simulink model "System_Theta_Space"  (R2019b)
settings: Solver=VariableStepAuto  StartTime=0.0  StopTime=10  FixedStep=.001  MaxStep=.001  RelTol=1e-6  EnableMultiTasking=on
values from neighbouring files (symbols this model uses):
  Kd = [75;75;75;40;1;1]    [SimRun_ThetaSpace.m]
  Ki = [0;500;300;300;0;0]    [SimRun_ThetaSpace.m]
  Kp = [500;500;500;300;10;10]    [SimRun_ThetaSpace.m]
undefined symbols (not defined in the file or in its folder): DiscIntNeverNeededParam
(part 1 of 4)
settings Model: Creator=Andrew Petruska  LastModifiedBy=Andrew Petruska
settings DataIOCC: ReturnWorkspaceOutputs=off
settings OptimizationCC: LifeSpan=inf
settings DebuggingCC: SFUnexpectedBacktrackingDiag=warning  SFNoUnconditionalDefaultTransitionDiag=warning  ArithmeticOperatorsInVariantConditions=warning
settings SFSimCC: SimUseLocalCustomCode=off  CustomCodeUndefinedFunction=UseInterfaceOnly
settings RTWCC: RTWUseLocalCustomCode=off
settings CodeAppCC: StateflowObjectComments=on
settings GRTTargetCC: TargetLangStandard=C89/C90 (ANSI)  GeneratePreprocessorConditionals=Disable all
settings ConfigComp: CovMetricSettings=dw  CovHtmlReporting=on  CovSaveCumulativeToWorkspaceVar=on  CovSaveSingleToWorkspaceVar=on  CovExternalEMLEnable=off

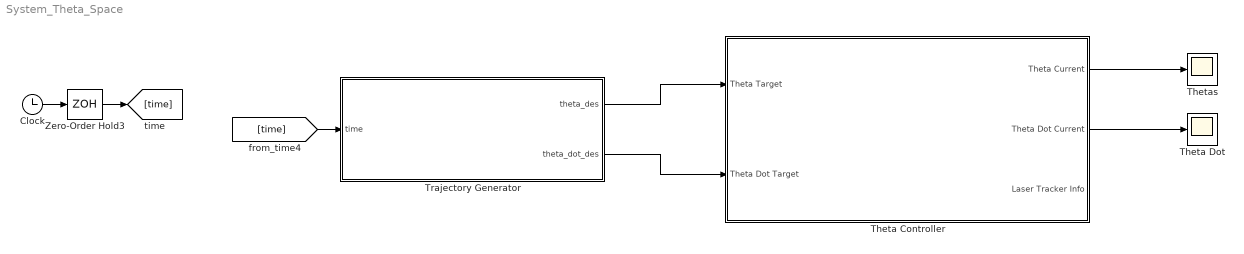
== system System_Theta_Space ==
  Clock : Clock
  Theta Controller : Subsystem
  Theta Dot : Scope
  Thetas : Scope
  Trajectory Generator : MATLAB Function  TreatAsAtomicUnit=on
  Zero-Order Hold3 : ZeroOrderHold  SampleTime=0.001
  wires:
  Clock/1 -> Zero-Order Hold3/1
  Zero-Order Hold3/1 -> [time]
  [time] -> Trajectory Generator/1(time)
  Theta Controller/1(Theta Current) -> Thetas/1
  Theta Controller/2(Theta Dot Current) -> Theta Dot/1
  Trajectory Generator/1(theta_des) -> Theta Controller/1(Theta Target)
  Trajectory Generator/2(theta_dot_des) -> Theta Controller/2(Theta Dot Target)

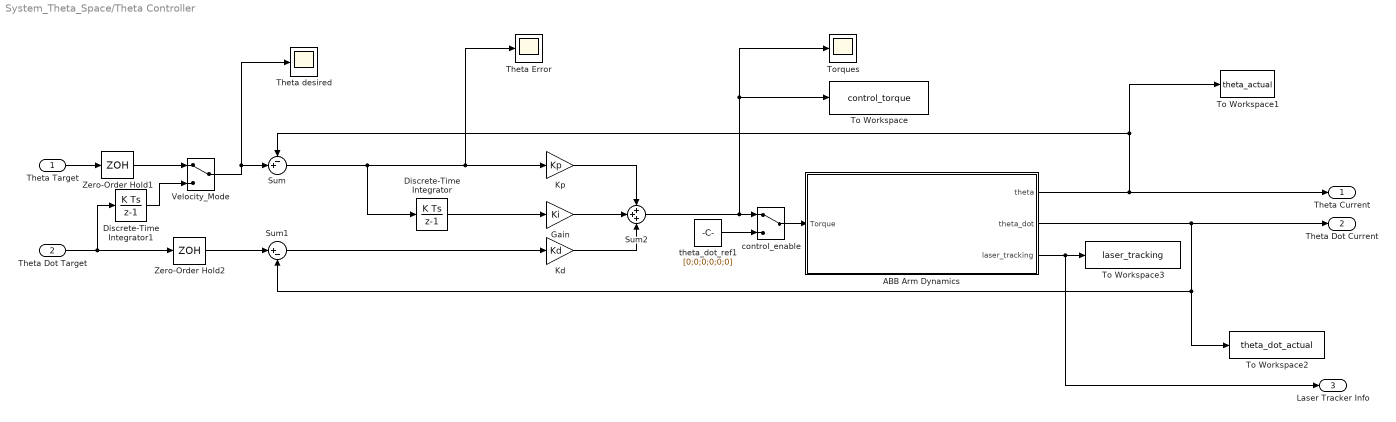
== system System_Theta_Space/Theta Controller ==
  Theta Target : Inport
  Theta Dot Target : Inport  Port=2
  ABB Arm Dynamics : Subsystem
  Discrete-Time Integrator : DiscreteIntegrator  gainval=1  SampleTime=-1  ICPrevOutput=DiscIntNeverNeededParam  ICPrevScaledInput=DiscIntNeverNeededParam
  Discrete-Time Integrator1 : DiscreteIntegrator  gainval=1  SampleTime=-1  ICPrevOutput=DiscIntNeverNeededParam  ICPrevScaledInput=DiscIntNeverNeededParam
  Gain : Gain  Gain=Ki
  Kd : Gain  Gain=Kd
  Kp : Gain  Gain=Kp
  Sum : Sum  Inputs=-+|
  Sum1 : Sum  Inputs=|+-
  Sum2 : Sum  Inputs=+++
  Theta Error : Scope
  Theta desired : Scope
  To Workspace : ToWorkspace  VariableName=control_torque  SaveFormat=Structure With Time  SampleTime=-1
  To Workspace1 : ToWorkspace  VariableName=theta_actual  SaveFormat=Structure With Time  SampleTime=-1
  To Workspace2 : ToWorkspace  VariableName=theta_dot_actual  SaveFormat=Structure With Time  SampleTime=-1
  To Workspace3 : ToWorkspace  VariableName=laser_tracking  SaveFormat=Structure With Time  SampleTime=-1
  Torques : Scope
  Velocity_Mode : ManualSwitch
  Zero-Order Hold1 : ZeroOrderHold  SampleTime=0.001
  Zero-Order Hold2 : ZeroOrderHold  SampleTime=0.001
  control_enable : ManualSwitch
  theta_dot_ref1 : Constant  Value=[0;0;0;0;0;0]
  Theta Current : Outport
  Theta Dot Current : Outport  Port=2
  Laser Tracker Info : Outport  Port=3
  wires:
  control_enable/1 -> ABB Arm Dynamics/1(Torque)
  ABB Arm Dynamics/1(theta) -> Sum/1, To Workspace1/1, Theta Current/1
  Sum/1 -> Discrete-Time Integrator/1, Theta Error/1, Kp/1
  ABB Arm Dynamics/2(theta_dot) -> Sum1/2, To Workspace2/1, Theta Dot Current/1
  Sum2/1 -> To Workspace/1, Torques/1, control_enable/1
  Discrete-Time Integrator/1 -> Gain/1
  theta_dot_ref1/1 -> control_enable/2
  ABB Arm Dynamics/3(laser_tracking) -> Laser Tracker Info/1, To Workspace3/1
  Sum1/1 -> Kd/1
  Kp/1 -> Sum2/1
  Gain/1 -> Sum2/2
  Kd/1 -> Sum2/3
  Theta Target/1 -> Zero-Order Hold1/1
  Theta Dot Target/1 -> Discrete-Time Integrator1/1, Zero-Order Hold2/1
  Zero-Order Hold2/1 -> Sum1/1
  Velocity_Mode/1 -> Theta desired/1, Sum/2
  Zero-Order Hold1/1 -> Velocity_Mode/1
  Discrete-Time Integrator1/1 -> Velocity_Mode/2

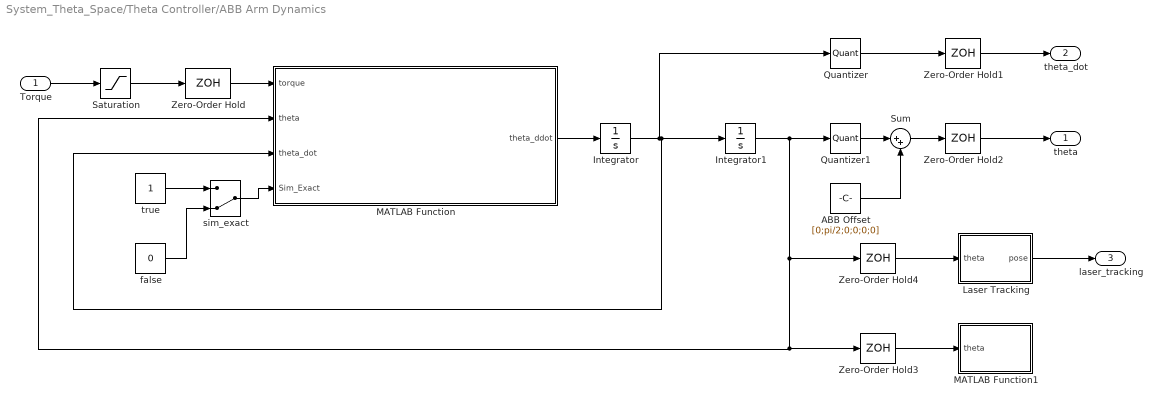
== system System_Theta_Space/Theta Controller/ABB Arm Dynamics ==
  Torque : Inport
  ABB Offset : Constant  Value=[0;pi/2;0;0;0;0]
  Integrator : Integrator  InitialCondition=zeros(6,1)
  Integrator1 : Integrator  InitialCondition=zeros(6,1)
  Laser Tracking : MATLAB Function  TreatAsAtomicUnit=on
  MATLAB Function : MATLAB Function  TreatAsAtomicUnit=on
  MATLAB Function1 : MATLAB Function  TreatAsAtomicUnit=on
  Quantizer : Quantizer  QuantizationInterval=1/2^32
  Quantizer1 : Quantizer  QuantizationInterval=1/2^32
  Saturation : Saturate  UpperLimit=350  LowerLimit=-350
  Sum : Sum  Inputs=|++
  Zero-Order Hold{,1..2,4} (4 alike) : ZeroOrderHold  SampleTime=0.001
  Zero-Order Hold3 : ZeroOrderHold  SampleTime=.05
  false : Constant  Value=0
  sim_exact : ManualSwitch  CurrentSetting=0
  true : Constant
  theta : Outport
  theta_dot : Outport  Port=2
  laser_tracking : Outport  Port=3
  wires:
  Torque/1 -> Saturation/1
  MATLAB Function/1(theta_ddot) -> Integrator/1
  Integrator/1 -> Quantizer/1, MATLAB Function/3(theta_dot), Integrator1/1
  Zero-Order Hold/1 -> MATLAB Function/1(torque)
  Quantizer/1 -> Zero-Order Hold1/1
  Zero-Order Hold1/1 -> theta_dot/1
  Zero-Order Hold2/1 -> theta/1
  Integrator1/1 -> Quantizer1/1, MATLAB Function/2(theta), Zero-Order Hold3/1, Zero-Order Hold4/1
  Zero-Order Hold3/1 -> MATLAB Function1/1(theta)
  Sum/1 -> Zero-Order Hold2/1
  Quantizer1/1 -> Sum/1
  ABB Offset/1 -> Sum/2
  Laser Tracking/1(pose) -> laser_tracking/1
  Saturation/1 -> Zero-Order Hold/1
  Zero-Order Hold4/1 -> Laser Tracking/1(theta)
  sim_exact/1 -> MATLAB Function/4(Sim_Exact)
  true/1 -> sim_exact/1
  false/1 -> sim_exact/2

== matlab function System_Theta_Space/Theta Controller/ABB Arm Dynamics/MATLAB Function1 ==
  data: theta input
function drawArm(theta)
%#codegen
coder.extrinsic('evalin');
coder.extrinsic('load');
persistent figNum axisHandel Sim_Exact points3D drawCSM sizeCSM;

if isempty(Sim_Exact)
    Sim_Exact = evalin('base','Sim_Exact');
    sizeCSM = 1;
    sizeCSM = evalin('base','sizeCSM');
    drawCSM = evalin('base','drawCSM');
    points3D = zeros(sizeCSM,3,'double');
    
    if drawCSM
        %a.points3D = zeros(sizeCSM,3,'double');
        a = struct('points3D',points3D);
        a = load('points3D.mat','points3D');
        points3D = a.points3D;
    end
end

th1 = theta(1);
th2 = theta(2);
th3 = theta(3);
th4 = theta(4);
th5 = theta(5);
th6 = theta(6);

if(Sim_Exact)
    
    T06 = [ sin(th6)*(cos(th4)*sin(th1) + sin(th4)*(cos(th1)*sin(th2)*sin(th3) - cos(th1)*cos(th2)*cos(th3))) + cos(th6)*(cos(th5)*(sin(th1)*sin(th4) - cos(th4)*(cos(th1)*sin(th2)*sin(th3) - cos(th1)*cos(th2)*cos(th3))) - sin(th5)*(cos(th1)*cos(th2)*sin(th3) + cos(th1)*cos(th3)*sin(th2))), cos(th6)*(cos(th4)*sin(th1) + sin(th4)*(cos(th1)*sin(th2)*sin(th3) - cos(th1)*cos(th2)*cos(th3))) - sin(th6)*(cos(th5)*(sin(th1)*sin(th4) - cos(th4)*(cos(th1)*sin(th2)*sin(th3) - cos(th1)*cos(th2)*cos(th3))) - sin(th5)*(cos(th1)*cos(th2)*sin(th3) + cos(th1)*cos(th3)*sin(th2))), - sin(th5)*(sin(th1)*sin(th4) - cos(th4)*(cos(th1)*sin(th2)*sin(th3) - cos(th1)*cos(th2)*cos(th3))) - cos(th5)*(cos(th1)*cos(th2)*sin(th3) + cos(th1)*cos(th3)*sin(th2)), (27*cos(th1)*cos(th2))/100 - (9*sin(th5)*(sin(th1)*sin(th4) - cos(th4)*(cos(th1)*sin(th2)*sin(th3) - cos(th1)*cos(th2)*cos(th3))))/125 - (9*cos(th5)*(cos(th1)*cos(th2)*sin(th3) + cos(th1)*cos(th3)*sin(th2)))/125 - (7*cos(th1)*sin(th2)*sin(th3))/100 + (7*cos(th1)*cos(th2)*cos(th3))/100 - (151*cos(th1)*cos(th2)*sin(th3))/500 - (151*cos(th1)*cos(th3)*sin(th2))/500;
        - sin(th6)*(cos(th1)*cos(th4) - sin(th4)*(sin(th1)*sin(th2)*sin(th3) - cos(th2)*cos(th3)*sin(th1))) - cos(th6)*(cos(th5)*(cos(th1)*sin(th4) + cos(th4)*(sin(th1)*sin(th2)*sin(th3) - cos(th2)*cos(th3)*sin(th1))) + sin(th5)*(cos(th2)*sin(th1)*sin(th3) + cos(th3)*sin(th1)*sin(th2))), sin(th6)*(cos(th5)*(cos(th1)*sin(th4) + cos(th4)*(sin(th1)*sin(th2)*sin(th3) - cos(th2)*cos(th3)*sin(th1))) + sin(th5)*(cos(th2)*sin(th1)*sin(th3) + cos(th3)*sin(th1)*sin(th2))) - cos(th6)*(cos(th1)*cos(th4) - sin(th4)*(sin(th1)*sin(th2)*sin(th3) - cos(th2)*cos(th3)*sin(th1))), sin(th5)*(cos(th1)*sin(th4) + cos(th4)*(sin(th1)*sin(th2)*sin(th3) - cos(th2)*cos(th3)*sin(th1))) - cos(th5)*(cos(th2)*sin(th1)*sin(th3) + cos(th3)*sin(th1)*sin(th2)), (27*cos(th2)*sin(th1))/100 + (9*sin(th5)*(cos(th1)*sin(th4) + cos(th4)*(sin(th1)*sin(th2)*sin(th3) - cos(th2)*cos(th3)*sin(th1))))/125 - (9*cos(th5)*(cos(th2)*sin(th1)*sin(th3) + cos(th3)*sin(th1)*sin(th2)))/125 - (151*cos(th2)*sin(th1)*sin(th3))/500 - (151*cos(th3)*sin(th1)*sin(th2))/500 - (7*sin(th1)*sin(th2)*sin(th3))/100 + (7*cos(th2)*cos(th3)*sin(th1))/100;
        sin(th4)*sin(th6)*(cos(th2)*sin(th3) + cos(th3)*sin(th2)) - cos(th6)*(sin(th5)*(cos(th2)*cos(th3) - sin(th2)*sin(th3)) + cos(th4)*cos(th5)*(cos(th2)*sin(th3) + cos(th3)*sin(th2))), sin(th6)*(sin(th5)*(cos(th2)*cos(th3) - sin(th2)*sin(th3)) + cos(th4)*cos(th5)*(cos(th2)*sin(th3) + cos(th3)*sin(th2))) + cos(th6)*sin(th4)*(cos(th2)*sin(th3) + cos(th3)*sin(th2)), cos(th4)*sin(th5)*(cos(th2)*sin(th3) + cos(th3)*sin(th2)) - cos(th5)*(cos(th2)*cos(th3) - sin(th2)*sin(th3)), (151*sin(th2)*sin(th3))/500 - (151*cos(th2)*cos(th3))/500 - (7*cos(th2)*sin(th3))/100 - (7*cos(th3)*sin(th2))/100 - (27*sin(th2))/100 - (9*cos(th5)*(cos(th2)*cos(th3) - sin(th2)*sin(th3)))/125 + (9*cos(th4)*sin(th5)*(cos(th2)*sin(th3) + cos(th3)*sin(th2)))/125 + 29/100;
        0, 0, 0, 1];
    
    P1 =[ 0
        0
        0.29];
    P2 = [ 0.27*cos(th1)*cos(th2);
        0.27*cos(th2)*sin(th1);
        0.29 - 0.27*sin(th2)];
    P3 = [ 0.27*cos(th1)*cos(th2) - 0.07*cos(th1)*sin(th2)*sin(th3) + 0.07*cos(th1)*cos(th2)*cos(th3);
        0.27*cos(th2)*sin(th1) - 0.07*sin(th1)*sin(th2)*sin(th3) + 0.07*cos(th2)*cos(th3)*sin(th1);
        0.29 - 0.07*cos(th2)*sin(th3) - 0.07*cos(th3)*sin(th2) - 0.27*sin(th2)];
    
    P4 = [ 0.27*cos(th1)*cos(th2) - 0.07*cos(th1)*sin(th2)*sin(th3) + 0.07*cos(th1)*cos(th2)*cos(th3) - 0.302*cos(th1)*cos(th2)*sin(th3) - 0.302*cos(th1)*cos(th3)*sin(th2);
        0.27*cos(th2)*sin(th1) - 0.302*cos(th2)*sin(th1)*sin(th3) - 0.302*cos(th3)*sin(th1)*sin(th2) - 0.07*sin(th1)*sin(th2)*sin(th3) + 0.07*cos(th2)*cos(th3)*sin(th1);
        0.302*sin(th2)*sin(th3) - 0.302*cos(th2)*cos(th3) - 0.07*cos(th2)*sin(th3) - 0.07*cos(th3)*sin(th2) - 0.27*sin(th2) + 0.29];
    P5 = [ 0.27*cos(th1)*cos(th2) - 0.07*cos(th1)*sin(th2)*sin(th3) + 0.07*cos(th1)*cos(th2)*cos(th3) - 0.302*cos(th1)*cos(th2)*sin(th3) - 0.302*cos(th1)*cos(th3)*sin(th2)
        0.27*cos(th2)*sin(th1) - 0.302*cos(th2)*sin(th1)*sin(th3) - 0.302*cos(th3)*sin(th1)*sin(th2) - 0.07*sin(th1)*sin(th2)*sin(th3) + 0.07*cos(th2)*cos(th3)*sin(th1)
        0.302*sin(th2)*sin(th3) - 0.302*cos(th2)*cos(th3) - 0.07*cos(th2)*sin(th3) - 0.07*cos(th3)*sin(th2) - 0.27*sin(th2) + 0.29];
    
    P6 =[ 0.27*cos(th1)*cos(th2) - 0.07*cos(th1)*sin(th2)*sin(th3) - 0.072*sin(th1)*sin(th4)*sin(th5) + 0.07*cos(th1)*cos(th2)*cos(th3) - 0.302*cos(th1)*cos(th2)*sin(th3) - 0.302*cos(th1)*cos(th3)*sin(th2) - 0.072*cos(th1)*cos(th2)*cos(th5)*sin(th3) - 0.072*cos(th1)*cos(th3)*cos(th5)*sin(th2) - 0.072*cos(th1)*cos(th2)*cos(th3)*cos(th4)*sin(th5) + 0.072*cos(th1)*cos(th4)*sin(th2)*sin(th3)*sin(th5);
        0.27*cos(th2)*sin(th1) - 0.302*cos(th2)*sin(th1)*sin(th3) - 0.302*cos(th3)*sin(th1)*sin(th2) + 0.072*cos(th1)*sin(th4)*sin(th5) - 0.07*sin(th1)*sin(th2)*sin(th3) + 0.07*cos(th2)*cos(th3)*sin(th1) - 0.072*cos(th2)*cos(th5)*sin(th1)*sin(th3) - 0.072*cos(th3)*cos(th5)*sin(th1)*sin(th2) - 0.072*cos(th2)*cos(th3)*cos(th4)*sin(th1)*sin(th5) + 0.072*cos(th4)*sin(th1)*sin(th2)*sin(th3)*sin(th5);
        0.302*sin(th2)*sin(th3) - 0.302*cos(th2)*cos(th3) - 0.07*cos(th2)*sin(th3) - 0.07*cos(th3)*sin(th2) - 0.27*sin(th2) + 0.072*cos(th5)*sin(th2)*sin(th3) - 0.072*cos(th2)*cos(th3)*cos(th5) + 0.072*cos(th2)*cos(th4)*sin(th3)*sin(th5) + 0.072*cos(th3)*cos(th4)*sin(th2)*sin(th5) + 0.29];
    
else
    
    T06 = [ sin(th6)*(cos(th4)*sin(th1) + sin(th4)*(cos(th1)*sin(th2)*sin(th3) - cos(th1)*cos(th2)*cos(th3))) + cos(th6)*(cos(th5)*(sin(th1)*sin(th4) - cos(th4)*(cos(th1)*sin(th2)*sin(th3) - cos(th1)*cos(th2)*cos(th3))) - sin(th5)*(cos(th1)*cos(th2)*sin(th3) + cos(th1)*cos(th3)*sin(th2))), cos(th6)*(cos(th4)*sin(th1) + sin(th4)*(cos(th1)*sin(th2)*sin(th3) - cos(th1)*cos(th2)*cos(th3))) - sin(th6)*(cos(th5)*(sin(th1)*sin(th4) - cos(th4)*(cos(th1)*sin(th2)*sin(th3) - cos(th1)*cos(th2)*cos(th3))) - sin(th5)*(cos(th1)*cos(th2)*sin(th3) + cos(th1)*cos(th3)*sin(th2))), - sin(th5)*(sin(th1)*sin(th4) - cos(th4)*(cos(th1)*sin(th2)*sin(th3) - cos(th1)*cos(th2)*cos(th3))) - cos(th5)*(cos(th1)*cos(th2)*sin(th3) + cos(th1)*cos(th3)*sin(th2)), (151838081588107*cos(th1)*cos(th2))/562949953421312 - (123928564092639*sin(th1))/72057594037927936 - (7184037743251309*cos(th1))/36893488147419103232 - (7330531551818703*cos(th4)*sin(th1))/36893488147419103232 - (5489399374888815*sin(th1)*sin(th4))/9223372036854775808 + (970893499285375*cos(th5)*(sin(th1)*sin(th4) - cos(th4)*(cos(th1)*sin(th2)*sin(th3) - cos(th1)*cos(th2)*cos(th3))))/9223372036854775808 - (5192391675427195*sin(th5)*(sin(th1)*sin(th4) - cos(th4)*(cos(th1)*sin(th2)*sin(th3) - cos(th1)*cos(th2)*cos(th3))))/72057594037927936 + (1663072680156839*sin(th6)*(cos(th4)*sin(th1) + sin(th4)*(cos(th1)*sin(th2)*sin(th3) - cos(th1)*cos(th2)*cos(th3))))/2305843009213693952 + (1663072680156839*cos(th6)*(cos(th5)*(sin(th1)*sin(th4) - cos(th4)*(cos(th1)*sin(th2)*sin(th3) - cos(th1)*cos(th2)*cos(th3))) - sin(th5)*(cos(th1)*cos(th2)*sin(th3) + cos(th1)*cos(th3)*sin(th2))))/2305843009213693952 + (5489399374888815*cos(th4)*(cos(th1)*sin(th2)*sin(th3) - cos(th1)*cos(th2)*cos(th3)))/9223372036854775808 - (5192391675427195*cos(th5)*(cos(th1)*cos(th2)*sin(th3) + cos(th1)*cos(th3)*sin(th2)))/72057594037927936 - (7330531551818703*sin(th4)*(cos(th1)*sin(th2)*sin(th3) - cos(th1)*cos(th2)*cos(th3)))/36893488147419103232 - (970893499285375*sin(th5)*(cos(th1)*cos(th2)*sin(th3) + cos(th1)*cos(th3)*sin(th2)))/9223372036854775808 - (1259578569946919*cos(th1)*sin(th2)*sin(th3))/18014398509481984 + (1259578569946919*cos(th1)*cos(th2)*cos(th3))/18014398509481984 - (5430591396830085*cos(th1)*cos(th2)*sin(th3))/18014398509481984 - (5430591396830085*cos(th1)*cos(th3)*sin(th2))/18014398509481984;
        - sin(th6)*(cos(th1)*cos(th4) - sin(th4)*(sin(th1)*sin(th2)*sin(th3) - cos(th2)*cos(th3)*sin(th1))) - cos(th6)*(cos(th5)*(cos(th1)*sin(th4) + cos(th4)*(sin(th1)*sin(th2)*sin(th3) - cos(th2)*cos(th3)*sin(th1))) + sin(th5)*(cos(th2)*sin(th1)*sin(th3) + cos(th3)*sin(th1)*sin(th2))), sin(th6)*(cos(th5)*(cos(th1)*sin(th4) + cos(th4)*(sin(th1)*sin(th2)*sin(th3) - cos(th2)*cos(th3)*sin(th1))) + sin(th5)*(cos(th2)*sin(th1)*sin(th3) + cos(th3)*sin(th1)*sin(th2))) - cos(th6)*(cos(th1)*cos(th4) - sin(th4)*(sin(th1)*sin(th2)*sin(th3) - cos(th2)*cos(th3)*sin(th1))), sin(th5)*(cos(th1)*sin(th4) + cos(th4)*(sin(th1)*sin(th2)*sin(th3) - cos(th2)*cos(th3)*sin(th1))) - cos(th5)*(cos(th2)*sin(th1)*sin(th3) + cos(th3)*sin(th1)*sin(th2)), (123928564092639*cos(th1))/72057594037927936 - (7184037743251309*sin(th1))/36893488147419103232 + (7330531551818703*cos(th1)*cos(th4))/36893488147419103232 + (151838081588107*cos(th2)*sin(th1))/562949953421312 + (5489399374888815*cos(th1)*sin(th4))/9223372036854775808 - (970893499285375*cos(th5)*(cos(th1)*sin(th4) + cos(th4)*(sin(th1)*sin(th2)*sin(th3) - cos(th2)*cos(th3)*sin(th1))))/9223372036854775808 + (5192391675427195*sin(th5)*(cos(th1)*sin(th4) + cos(th4)*(sin(th1)*sin(th2)*sin(th3) - cos(th2)*cos(th3)*sin(th1))))/72057594037927936 - (1663072680156839*sin(th6)*(cos(th1)*cos(th4) - sin(th4)*(sin(th1)*sin(th2)*sin(th3) - cos(th2)*cos(th3)*sin(th1))))/2305843009213693952 + (5489399374888815*cos(th4)*(sin(th1)*sin(th2)*sin(th3) - cos(th2)*cos(th3)*sin(th1)))/9223372036854775808 - (5192391675427195*cos(th5)*(cos(th2)*sin(th1)*sin(th3) + cos(th3)*sin(th1)*sin(th2)))/72057594037927936 - (1663072680156839*cos(th6)*(cos(th5)*(cos(th1)*sin(th4) + cos(th4)*(sin(th1)*sin(th2)*sin(th3) - cos(th2)*cos(th3)*sin(th1))) + sin(th5)*(cos(th2)*sin(th1)*sin(th3) + cos(th3)*sin(th1)*sin(th2))))/2305843009213693952 - (7330531551818703*sin(th4)*(sin(th1)*sin(th2)*sin(th3) - cos(th2)*cos(th3)*sin(th1)))/36893488147419103232 - (970893499285375*sin(th5)*(cos(th2)*sin(th1)*sin(th3) + cos(th3)*sin(th1)*sin(th2)))/9223372036854775808 - (5430591396830085*cos(th2)*sin(th1)*sin(th3))/18014398509481984 - (5430591396830085*cos(th3)*sin(th1)*sin(th2))/18014398509481984 - (1259578569946919*sin(th1)*sin(th2)*sin(th3))/18014398509481984 + (1259578569946919*cos(th2)*cos(th3)*sin(th1))/18014398509481984;
        sin(th4)*sin(th6)*(cos(th2)*sin(th3) + cos(th3)*sin(th2)) - cos(th6)*(sin(th5)*(cos(th2)*cos(th3) - sin(th2)*sin(th3)) + cos(th4)*cos(th5)*(cos(th2)*sin(th3) + cos(th3)*sin(th2))), sin(th6)*(sin(th5)*(cos(th2)*cos(th3) - sin(th2)*sin(th3)) + cos(th4)*cos(th5)*(cos(th2)*sin(th3) + cos(th3)*sin(th2))) + cos(th6)*sin(th4)*(cos(th2)*sin(th3) + cos(th3)*sin(th2)), cos(th4)*sin(th5)*(cos(th2)*sin(th3) + cos(th3)*sin(th2)) - cos(th5)*(cos(th2)*cos(th3) - sin(th2)*sin(th3)), (5430591396830085*sin(th2)*sin(th3))/18014398509481984 - (5430591396830085*cos(th2)*cos(th3))/18014398509481984 - (1259578569946919*cos(th2)*sin(th3))/18014398509481984 - (1259578569946919*cos(th3)*sin(th2))/18014398509481984 - (1663072680156839*cos(th6)*(sin(th5)*(cos(th2)*cos(th3) - sin(th2)*sin(th3)) + cos(th4)*cos(th5)*(cos(th2)*sin(th3) + cos(th3)*sin(th2))))/2305843009213693952 - (151838081588107*sin(th2))/562949953421312 + (5489399374888815*cos(th4)*(cos(th2)*sin(th3) + cos(th3)*sin(th2)))/9223372036854775808 - (5192391675427195*cos(th5)*(cos(th2)*cos(th3) - sin(th2)*sin(th3)))/72057594037927936 - (7330531551818703*sin(th4)*(cos(th2)*sin(th3) + cos(th3)*sin(th2)))/36893488147419103232 - (970893499285375*sin(th5)*(cos(th2)*cos(th3) - sin(th2)*sin(th3)))/9223372036854775808 - (970893499285375*cos(th4)*cos(th5)*(cos(th2)*sin(th3) + cos(th3)*sin(th2)))/9223372036854775808 + (5192391675427195*cos(th4)*sin(th5)*(cos(th2)*sin(th3) + cos(th3)*sin(th2)))/72057594037927936 + (1663072680156839*sin(th4)*sin(th6)*(cos(th2)*sin(th3) + cos(th3)*sin(th2)))/2305843009213693952 + 325695105792877/1125899906842624;
        0, 0, 0, 1];
    P1 = [ -0.000194724*cos(th1);
        -0.000194724*sin(th1);
        0.289275];
    P2 =[ 0.269719*cos(th1)*cos(th2) - 0.000812193*sin(th1) - 0.000194724*cos(th1);
        0.000812193*cos(th1) - 0.000194724*sin(th1) + 0.269719*cos(th2)*sin(th1);
        0.289275 - 0.269719*sin(th2)];
    P3 =[ 0.269719*cos(th1)*cos(th2) - 0.00171985*sin(th1) - 0.000194724*cos(th1) - 0.0699207*cos(th1)*sin(th2)*sin(th3) + 0.0699207*cos(th1)*cos(th2)*cos(th3);
        0.00171985*cos(th1) - 0.000194724*sin(th1) + 0.269719*cos(th2)*sin(th1) - 0.0699207*sin(th1)*sin(th2)*sin(th3) + 0.0699207*cos(th2)*cos(th3)*sin(th1);
        0.289275 - 0.0699207*cos(th2)*sin(th3) - 0.0699207*cos(th3)*sin(th2) - 0.269719*sin(th2)];
    
    P4 =[ 0.269719*cos(th1)*cos(th2) - 0.00171985*sin(th1) - 0.000194724*cos(th1) - 0.000595162*sin(th1)*sin(th4) - 0.0699207*cos(th1)*sin(th2)*sin(th3) + 0.0699207*cos(th1)*cos(th2)*cos(th3) - 0.301458*cos(th1)*cos(th2)*sin(th3) - 0.301458*cos(th1)*cos(th3)*sin(th2) - 0.000595162*cos(th1)*cos(th2)*cos(th3)*cos(th4) + 0.000595162*cos(th1)*cos(th4)*sin(th2)*sin(th3);
        0.00171985*cos(th1) - 0.000194724*sin(th1) + 0.269719*cos(th2)*sin(th1) + 0.000595162*cos(th1)*sin(th4) - 0.301458*cos(th2)*sin(th1)*sin(th3) - 0.301458*cos(th3)*sin(th1)*sin(th2) - 0.0699207*sin(th1)*sin(th2)*sin(th3) + 0.0699207*cos(th2)*cos(th3)*sin(th1) - 0.000595162*cos(th2)*cos(th3)*cos(th4)*sin(th1) + 0.000595162*cos(th4)*sin(th1)*sin(th2)*sin(th3);
        0.301458*sin(th2)*sin(th3) - 0.301458*cos(th2)*cos(th3) - 0.0699207*cos(th2)*sin(th3) - 0.0699207*cos(th3)*sin(th2) - 0.269719*sin(th2) + 0.000595162*cos(th2)*cos(th4)*sin(th3) + 0.000595162*cos(th3)*cos(th4)*sin(th2) + 0.289275];
    
    P5 = [ 0.269719*cos(th1)*cos(th2) - 0.00171985*sin(th1) - 0.000194724*cos(th1) - 0.000198694*cos(th4)*sin(th1) - 0.000595162*sin(th1)*sin(th4) - 0.0699207*cos(th1)*sin(th2)*sin(th3) + 0.000105264*cos(th5)*sin(th1)*sin(th4) + 0.0699207*cos(th1)*cos(th2)*cos(th3) - 0.301458*cos(th1)*cos(th2)*sin(th3) - 0.301458*cos(th1)*cos(th3)*sin(th2) - 0.000595162*cos(th1)*cos(th2)*cos(th3)*cos(th4) + 0.000198694*cos(th1)*cos(th2)*cos(th3)*sin(th4) + 0.000595162*cos(th1)*cos(th4)*sin(th2)*sin(th3) - 0.000105264*cos(th1)*cos(th2)*sin(th3)*sin(th5) - 0.000105264*cos(th1)*cos(th3)*sin(th2)*sin(th5) - 0.000198694*cos(th1)*sin(th2)*sin(th3)*sin(th4) + 0.000105264*cos(th1)*cos(th2)*cos(th3)*cos(th4)*cos(th5) - 0.000105264*cos(th1)*cos(th4)*cos(th5)*sin(th2)*sin(th3);
        0.00171985*cos(th1) - 0.000194724*sin(th1) + 0.000198694*cos(th1)*cos(th4) + 0.269719*cos(th2)*sin(th1) + 0.000595162*cos(th1)*sin(th4) - 0.301458*cos(th2)*sin(th1)*sin(th3) - 0.301458*cos(th3)*sin(th1)*sin(th2) - 0.0699207*sin(th1)*sin(th2)*sin(th3) + 0.0699207*cos(th2)*cos(th3)*sin(th1) - 0.000105264*cos(th1)*cos(th5)*sin(th4) - 0.000595162*cos(th2)*cos(th3)*cos(th4)*sin(th1) + 0.000198694*cos(th2)*cos(th3)*sin(th1)*sin(th4) + 0.000595162*cos(th4)*sin(th1)*sin(th2)*sin(th3) - 0.000105264*cos(th2)*sin(th1)*sin(th3)*sin(th5) - 0.000105264*cos(th3)*sin(th1)*sin(th2)*sin(th5) - 0.000198694*sin(th1)*sin(th2)*sin(th3)*sin(th4) + 0.000105264*cos(th2)*cos(th3)*cos(th4)*cos(th5)*sin(th1) - 0.000105264*cos(th4)*cos(th5)*sin(th1)*sin(th2)*sin(th3);
        0.301458*sin(th2)*sin(th3) - 0.301458*cos(th2)*cos(th3) - 0.0699207*cos(th2)*sin(th3) - 0.0699207*cos(th3)*sin(th2) - 0.269719*sin(th2) - 0.000198694*cos(th2)*sin(th3)*sin(th4) - 0.000198694*cos(th3)*sin(th2)*sin(th4) + 0.000105264*sin(th2)*sin(th3)*sin(th5) + 0.000595162*cos(th2)*cos(th4)*sin(th3) + 0.000595162*cos(th3)*cos(th4)*sin(th2) - 0.000105264*cos(th2)*cos(th3)*sin(th5) - 0.000105264*cos(th2)*cos(th4)*cos(th5)*sin(th3) - 0.000105264*cos(th3)*cos(th4)*cos(th5)*sin(th2) + 0.289275];
    
    P6 =[ 0.269719*cos(th1)*cos(th2) - 0.00171985*sin(th1) - 0.000194724*cos(th1) - 0.000198694*cos(th4)*sin(th1) - 0.000595162*sin(th1)*sin(th4) - 0.0699207*cos(th1)*sin(th2)*sin(th3) + 0.000105264*cos(th5)*sin(th1)*sin(th4) + 0.000721243*cos(th4)*sin(th1)*sin(th6) - 0.0720589*sin(th1)*sin(th4)*sin(th5) + 0.0699207*cos(th1)*cos(th2)*cos(th3) - 0.301458*cos(th1)*cos(th2)*sin(th3) - 0.301458*cos(th1)*cos(th3)*sin(th2) - 0.000595162*cos(th1)*cos(th2)*cos(th3)*cos(th4) + 0.000198694*cos(th1)*cos(th2)*cos(th3)*sin(th4) - 0.0720589*cos(th1)*cos(th2)*cos(th5)*sin(th3) - 0.0720589*cos(th1)*cos(th3)*cos(th5)*sin(th2) + 0.000595162*cos(th1)*cos(th4)*sin(th2)*sin(th3) - 0.000105264*cos(th1)*cos(th2)*sin(th3)*sin(th5) - 0.000105264*cos(th1)*cos(th3)*sin(th2)*sin(th5) + 0.000721243*cos(th5)*cos(th6)*sin(th1)*sin(th4) - 0.000198694*cos(th1)*sin(th2)*sin(th3)*sin(th4) + 0.000105264*cos(th1)*cos(th2)*cos(th3)*cos(th4)*cos(th5) - 0.0720589*cos(th1)*cos(th2)*cos(th3)*cos(th4)*sin(th5) - 0.000105264*cos(th1)*cos(th4)*cos(th5)*sin(th2)*sin(th3) - 0.000721243*cos(th1)*cos(th2)*cos(th3)*sin(th4)*sin(th6) - 0.000721243*cos(th1)*cos(th2)*cos(th6)*sin(th3)*sin(th5) - 0.000721243*cos(th1)*cos(th3)*cos(th6)*sin(th2)*sin(th5) + 0.0720589*cos(th1)*cos(th4)*sin(th2)*sin(th3)*sin(th5) + 0.000721243*cos(th1)*sin(th2)*sin(th3)*sin(th4)*sin(th6) + 0.000721243*cos(th1)*cos(th2)*cos(th3)*cos(th4)*cos(th5)*cos(th6) - 0.000721243*cos(th1)*cos(th4)*cos(th5)*cos(th6)*sin(th2)*sin(th3);
        0.00171985*cos(th1) - 0.000194724*sin(th1) + 0.000198694*cos(th1)*cos(th4) + 0.269719*cos(th2)*sin(th1) + 0.000595162*cos(th1)*sin(th4) - 0.301458*cos(th2)*sin(th1)*sin(th3) - 0.301458*cos(th3)*sin(th1)*sin(th2) + 0.0720589*cos(th1)*sin(th4)*sin(th5) - 0.0699207*sin(th1)*sin(th2)*sin(th3) + 0.0699207*cos(th2)*cos(th3)*sin(th1) - 0.000105264*cos(th1)*cos(th5)*sin(th4) - 0.000721243*cos(th1)*cos(th4)*sin(th6) - 0.000595162*cos(th2)*cos(th3)*cos(th4)*sin(th1) - 0.000721243*cos(th1)*cos(th5)*cos(th6)*sin(th4) + 0.000198694*cos(th2)*cos(th3)*sin(th1)*sin(th4) - 0.0720589*cos(th2)*cos(th5)*sin(th1)*sin(th3) - 0.0720589*cos(th3)*cos(th5)*sin(th1)*sin(th2) + 0.000595162*cos(th4)*sin(th1)*sin(th2)*sin(th3) - 0.000105264*cos(th2)*sin(th1)*sin(th3)*sin(th5) - 0.000105264*cos(th3)*sin(th1)*sin(th2)*sin(th5) - 0.000198694*sin(th1)*sin(th2)*sin(th3)*sin(th4) + 0.000105264*cos(th2)*cos(th3)*cos(th4)*cos(th5)*sin(th1) - 0.0720589*cos(th2)*cos(th3)*cos(th4)*sin(th1)*sin(th5) - 0.000105264*cos(th4)*cos(th5)*sin(th1)*sin(th2)*sin(th3) - 0.000721243*cos(th2)*cos(th3)*sin(th1)*sin(th4)*sin(th6) - 0.000721243*cos(th2)*cos(th6)*sin(th1)*sin(th3)*sin(th5) - 0.000721243*cos(th3)*cos(th6)*sin(th1)*sin(th2)*sin(th5) + 0.0720589*cos(th4)*sin(th1)*sin(th2)*sin(th3)*sin(th5) + 0.000721243*sin(th1)*sin(th2)*sin(th3)*sin(th4)*sin(th6) + 0.000721243*cos(th2)*cos(th3)*cos(th4)*cos(th5)*cos(th6)*sin(th1) - 0.000721243*cos(th4)*cos(th5)*cos(th6)*sin(th1)*sin(th2)*sin(th3);
        0.301458*sin(th2)*sin(th3) - 0.301458*cos(th2)*cos(th3) - 0.0699207*cos(th2)*sin(th3) - 0.0699207*cos(th3)*sin(th2) - 0.269719*sin(th2) - 0.000198694*cos(th2)*sin(th3)*sin(th4) - 0.000198694*cos(th3)*sin(th2)*sin(th4) + 0.0720589*cos(th5)*sin(th2)*sin(th3) + 0.000105264*sin(th2)*sin(th3)*sin(th5) - 0.0720589*cos(th2)*cos(th3)*cos(th5) + 0.000595162*cos(th2)*cos(th4)*sin(th3) + 0.000595162*cos(th3)*cos(th4)*sin(th2) - 0.000105264*cos(th2)*cos(th3)*sin(th5) - 0.000105264*cos(th2)*cos(th4)*cos(th5)*sin(th3) - 0.000105264*cos(th3)*cos(th4)*cos(th5)*sin(th2) - 0.000721243*cos(th2)*cos(th3)*cos(th6)*sin(th5) + 0.0720589*cos(th2)*cos(th4)*sin(th3)*sin(th5) + 0.0720589*cos(th3)*cos(th4)*sin(th2)*sin(th5) + 0.000721243*cos(th2)*sin(th3)*sin(th4)*sin(th6) + 0.000721243*cos(th3)*sin(th2)*sin(th4)*sin(th6) + 0.000721243*cos(th6)*sin(th2)*sin(th3)*sin(th5) - 0.000721243*cos(th2)*cos(th4)*cos(th5)*cos(th6)*sin(th3) - 0.000721243*cos(th3)*cos(th4)*cos(th5)*cos(th6)*sin(th2) + 0.289275];
    
end


if isempty(figNum)
    figNum = figure(1);
    hold on;
    plot3([0;P1(1);P2(1);P3(1);P4(1);P5(1);P6(1)],...
        [0;P1(2);P2(2);P3(2);P4(2);P5(2);P6(2)],...
        [0;P1(3);P2(3);P3(3);P4(3);P5(3);P6(3)],'k','linewidth',2);
    axisHandel = gca;
    plot3([P6(1);P6(1)+T06(1,1)*.1],...
        [P6(2);P6(2)+T06(2,1)*.1],...
        [P6(3);P6(3)+T06(3,1)*.1],'r','Parent',axisHandel);
    plot3([P6(1);P6(1)+T06(1,2)*.1],...
        [P6(2);P6(2)+T06(2,2)*.1],...
        [P6(3);P6(3)+T06(3,2)*.1],'g','Parent',axisHandel);
    plot3([P6(1);P6(1)+T06(1,3)*.1],...
        [P6(2);P6(2)+T06(2,3)*.1],...
        [P6(3);P6(3)+T06(3,3)*.1],'b','Parent',axisHandel);
    if drawCSM
    plot3(points3D(:,1),points3D(:,2),points3D(:,3),'m','Parent',axisHandel);
    end
    hold off;
    axis([-.75 .75 -.75 .75 -.4 .75]);
    axisHandel = gca;
else
    plot3([0;P1(1);P2(1);P3(1);P4(1);P5(1);P6(1)],...
        [0;P1(2);P2(2);P3(2);P4(2);P5(2);P6(2)],...
        [0;P1(3);P2(3);P3(3);P4(3);P5(3);P6(3)],'k','linewidth',2,'Parent',axisHandel);
    hold on;
    plot3([P6(1);P6(1)+T06(1,1)*.1],...
        [P6(2);P6(2)+T06(2,1)*.1],...
        [P6(3);P6(3)+T06(3,1)*.1],'r','Parent',axisHandel);
    plot3([P6(1);P6(1)+T06(1,2)*.1],...
        [P6(2);P6(2)+T06(2,2)*.1],...
        [P6(3);P6(3)+T06(3,2)*.1],'g','Parent',axisHandel);
    plot3([P6(1);P6(1)+T06(1,3)*.1],...
        [P6(2);P6(2)+T06(2,3)*.1],...
        [P6(3);P6(3)+T06(3,3)*.1],'b','Parent',axisHandel);
    if drawCSM
        plot3(points3D(:,1),points3D(:,2),points3D(:,3),'m','Parent',axisHandel);
    end
    hold off;
    axis([-.75 .75 -.75 .75 -.4 .75]);
end
